simulink library "generator_lib"  (Simulink 7.8)
settings: Solver=ode45  StartTime=0.0  StopTime=10.0  RelTol=1e-3
undefined symbols (not defined in the file): dfilt, DiscIntNeverNeededParam, fdesignblkfcn, gcbh, ph, Ts
libraries: simulink x91, rtio_opalrt_common x84, powerlib x51, simulink_extras x21, discretizing x14, rteventslib x14, dsparch4 x14, powerlib_extras x4
(part 9 of 10)

== system generator_lib/Generator_09112015/GenSet_4MVA_copy1mva/4MVA Generator with  Primary Controllers/Diesel Engine Speed & Voltage Control fast/Excitation/Damping kf.s / (tf.s +1) ==
  note: link disabled
  In : Inport
  1st-Order Discrete Filter : Subsystem  AncestorBlock=|  mask(Discrete 1st-Order Filter){FilterType=Highpass, Tc=damp(2), Ts=Ts, Initialize=on, Vac_Init=[0 0 60], Vdc_Init=damp(1)*v0(2)/damp(2), PlotResponse=off, param1=[1 500 0.1]}
      | powerlib_extras/Discrete 
      | Control Blocks/Discrete
      | 1st-Order
      | Discrete Filter
      mask prompts: FilterType "Filter Type:"; Tc "Time constant (s):"; Ts "Sample time:"; Initialize "Initialize filter states"; Vac_Init "AC initial input: [ Mag  Phase(degrees)  Freq(Hz) ]"; Vdc_Init "DC Initial input:"; PlotResponse "Plot filter response"; param1 "Frequency range(Hz) : [Start  End  Inc.]"
      mask init: same as generator_lib/1MVA Generator/GenSet_900kW_07232015/900kW Generator with  Primary Controllers/Diesel Engine Speed & Voltage Control fast/Excitation/Low Pass Filter 1 / (tr.s +1) (with IC)
      mask StyleString: popup(Lowpass|Highpass),edit,edit,checkbox,edit,edit,checkbox,edit
      mask CallbackString: |||p4=get_param(gcb,'Initialize');if strcmp(p4,'on');visible={'on','on','on','on','on','on','on',get_param(gcb,'PlotResponse')};else;visible={'on','on','on','on','off','off','on',get_param(gcb,'PlotResponse')};end;set_param(gcb,'MaskVisibilities',visible)|||p7=get_param(gcb,'PlotResponse');if strcmp(p7,'on');visible={'on','on','on','on',get_param(gcb,'Initialize'),get_param(gcb,'Initialize'),'on','on'};else;visible={'on','on','on','on',get_param(gcb,'Initialize'),get_param(gcb,'Initialize'),'on','off'};end;set_param(gcb,'MaskVisibilities',visible)|
      mask Display: plot(X,Y);
  Gain : Gain  Gain=damp(1)/damp(2)  SaturateOnIntegerOverflow=on  OutDataTypeStr=Inherit: Same as input  ParamDataTypeStr=Inherit: Same as input
  Out : Outport
  wires:
  1st-Order Discrete Filter/1(Out) -> Out/1
  Gain/1 -> 1st-Order Discrete Filter/1(In)
  In/1 -> Gain/1

== system generator_lib/Generator_09112015/GenSet_4MVA_copy1mva/4MVA Generator with  Primary Controllers/Diesel Engine Speed & Voltage Control fast/Excitation/Exciter  1 / (te.s + ke) ==
  note: link disabled
  In : Inport
  1st order Lowpass : Subsystem  AncestorBlock=|  mask(Discrete 1st-Order Filter){FilterType=Lowpass, Tc=exc(2)/exc(1), Ts=Ts, Initialize=on, Vac_Init=[0.0 0 60], Vdc_Init=v0(2), PlotResponse=off, param1=[1 500 0.1]}
      | powerlib_extras/Discrete 
      | Control Blocks/Discrete
      | 1st-Order
      | Discrete Filter
      mask prompts: FilterType "Filter Type:"; Tc "Time constant (s):"; Ts "Sample time:"; Initialize "Initialize filter states"; Vac_Init "AC initial input: [ Mag  Phase(degrees)  Freq(Hz) ]"; Vdc_Init "DC Initial input:"; PlotResponse "Plot filter response"; param1 "Frequency range(Hz) : [Start  End  Inc.]"
      mask init: same as generator_lib/1MVA Generator/GenSet_900kW_07232015/900kW Generator with  Primary Controllers/Diesel Engine Speed & Voltage Control fast/Excitation/Low Pass Filter 1 / (tr.s +1) (with IC)
      mask StyleString: popup(Lowpass|Highpass),edit,edit,checkbox,edit,edit,checkbox,edit
      mask CallbackString: |||p4=get_param(gcb,'Initialize');if strcmp(p4,'on');visible={'on','on','on','on','on','on','on',get_param(gcb,'PlotResponse')};else;visible={'on','on','on','on','off','off','on',get_param(gcb,'PlotResponse')};end;set_param(gcb,'MaskVisibilities',visible)|||p7=get_param(gcb,'PlotResponse');if strcmp(p7,'on');visible={'on','on','on','on',get_param(gcb,'Initialize'),get_param(gcb,'Initialize'),'on','on'};else;visible={'on','on','on','on',get_param(gcb,'Initialize'),get_param(gcb,'Initialize'),'on','off'};end;set_param(gcb,'MaskVisibilities',visible)|
      mask Display: plot(X,Y);
  Gain : Gain  Gain=1/exc(1)  SaturateOnIntegerOverflow=on  OutDataTypeStr=Inherit: Same as input  ParamDataTypeStr=Inherit: Same as input
  Out : Outport
  wires:
  Gain/1 -> 1st order Lowpass/1(In)
  In/1 -> Gain/1
  1st order Lowpass/1(Out) -> Out/1

== system generator_lib/Generator_09112015/GenSet_4MVA_copy1mva/4MVA Generator with  Primary Controllers/Diesel Engine Speed & Voltage Control fast/Excitation/Lead Lag Compensator tc.s+1 / tb.s+1 ==
  In1 : Inport
  Discrete State-Space : DiscreteStateSpace  A=Ad  B=Bd  C=Cd  D=Dd  X0=x0d  SampleTime=Ts
  Out1 : Outport
  wires:
  In1/1 -> Discrete State-Space/1
  Discrete State-Space/1 -> Out1/1

== system generator_lib/Generator_09112015/GenSet_4MVA_copy1mva/4MVA Generator with  Primary Controllers/Diesel Engine Speed & Voltage Control fast/Excitation/Low Pass Filter 1 / (tr.s +1) (with IC) ==
  In : Inport
  Discrete State-Space : DiscreteStateSpace  A=Ad  B=Bd  C=Cd  D=Dd  X0=x0d  SampleTime=Ts
  Out : Outport  InitialOutput=0
  wires:
  In/1 -> Discrete State-Space/1
  Discrete State-Space/1 -> Out/1

== system generator_lib/Generator_09112015/GenSet_4MVA_copy1mva/4MVA Generator with  Primary Controllers/Diesel Engine Speed & Voltage Control fast/Excitation/Main Regulator ka / (ta.s +1) ==
  note: link disabled
  In : Inport
  1st order Lowpass : Subsystem  AncestorBlock=|  mask(Discrete 1st-Order Filter){FilterType=Lowpass, Tc=reg(2), Ts=Ts, Initialize=on, Vac_Init=[0.0 0 60], Vdc_Init=exc(1)*v0(2), PlotResponse=off, param1=[1 500 0.1]}
      | powerlib_extras/Discrete 
      | Control Blocks/Discrete
      | 1st-Order
      | Discrete Filter
      mask prompts: FilterType "Filter Type:"; Tc "Time constant (s):"; Ts "Sample time:"; Initialize "Initialize filter states"; Vac_Init "AC initial input: [ Mag  Phase(degrees)  Freq(Hz) ]"; Vdc_Init "DC Initial input:"; PlotResponse "Plot filter response"; param1 "Frequency range(Hz) : [Start  End  Inc.]"
      mask init: same as generator_lib/1MVA Generator/GenSet_900kW_07232015/900kW Generator with  Primary Controllers/Diesel Engine Speed & Voltage Control fast/Excitation/Low Pass Filter 1 / (tr.s +1) (with IC)
      mask StyleString: popup(Lowpass|Highpass),edit,edit,checkbox,edit,edit,checkbox,edit
      mask CallbackString: |||p4=get_param(gcb,'Initialize');if strcmp(p4,'on');visible={'on','on','on','on','on','on','on',get_param(gcb,'PlotResponse')};else;visible={'on','on','on','on','off','off','on',get_param(gcb,'PlotResponse')};end;set_param(gcb,'MaskVisibilities',visible)|||p7=get_param(gcb,'PlotResponse');if strcmp(p7,'on');visible={'on','on','on','on',get_param(gcb,'Initialize'),get_param(gcb,'Initialize'),'on','on'};else;visible={'on','on','on','on',get_param(gcb,'Initialize'),get_param(gcb,'Initialize'),'on','off'};end;set_param(gcb,'MaskVisibilities',visible)|
      mask Display: plot(X,Y);
  Gain : Gain  Gain=reg(1)  SaturateOnIntegerOverflow=on  OutDataTypeStr=Inherit: Same as input  ParamDataTypeStr=Inherit: Same as input
  Out : Outport
  wires:
  1st order Lowpass/1(Out) -> Out/1
  In/1 -> Gain/1
  Gain/1 -> 1st order Lowpass/1(In)

== system generator_lib/Generator_09112015/GenSet_4MVA_copy1mva/4MVA Generator with  Primary Controllers/Diesel Engine Speed & Voltage Control fast/Excitation/proportional saturation ==
  Efd : Inport
  Vtf : Inport  Port=2
  Constant : Constant  Value=lim(3)
  Constant1 : Constant  Value=lim(1)
  Constant3 : Constant  Value=0
  Data Type  Conversion{,1..3} (4 alike) : DataTypeConversion  OutDataTypeStr=double  SaturateOnIntegerOverflow=on  RndMeth=Zero
  Logical Operator : Logic
  Logical Operator1 : Logic  Operator=NOT  Inputs=1
  Logical Operator2 : Logic  Operator=NOT  Inputs=1
  Product : Product  SaturateOnIntegerOverflow=on  InputSameDT=on  OutDataTypeStr=Inherit: Same as first input
  Product1 : Product  SaturateOnIntegerOverflow=on  InputSameDT=on  OutDataTypeStr=Inherit: Same as first input
  Product2 : Product  SaturateOnIntegerOverflow=on  InputSameDT=on  OutDataTypeStr=Inherit: Same as first input
  Relational Operator : RelationalOperator  Operator===  InputSameDT=on
  Relational Operator1 : RelationalOperator  Operator=<  InputSameDT=on
  Relational Operator2 : RelationalOperator  Operator=>  InputSameDT=on
  Sum : Sum  SaturateOnIntegerOverflow=on  InputSameDT=on  OutDataTypeStr=Inherit: Same as first input
  Sum1 : Sum  Inputs=+++  SaturateOnIntegerOverflow=on  InputSameDT=on  OutDataTypeStr=Inherit: Same as first input
  Vfdmax : Gain  Gain=lim(2)  SaturateOnIntegerOverflow=on  OutDataTypeStr=Inherit: Same as input  ParamDataTypeStr=Inherit: Same as input
  Vfdmax1 : Gain  Gain=lim(3)  SaturateOnIntegerOverflow=on  OutDataTypeStr=Inherit: Same as input  ParamDataTypeStr=Inherit: Same as input
  Ef : Outport  InitialOutput=0
  wires:
  Data Type  Conversion3/1 -> Vfdmax/1
  Relational Operator/1 -> Data Type  Conversion3/1
  Data Type  Conversion2/1 -> Product2/1
  Logical Operator2/1 -> Data Type  Conversion2/1
  Data Type  Conversion1/1 -> Product1/2
  Logical Operator1/1 -> Data Type  Conversion1/1
  Data Type  Conversion/1 -> Product/2
  Logical Operator/1 -> Data Type  Conversion/1
  Product1/1 -> Sum1/2
  Product2/1 -> Sum1/3
  Product/1 -> Sum1/1
  Sum1/1 -> Ef/1
  Efd/1 -> Product/1, Relational Operator1/1, Relational Operator2/1
  Constant1/1 -> Product1/1, Relational Operator2/2
  Relational Operator1/1 -> Logical Operator/2, Logical Operator2/1
  Relational Operator2/1 -> Logical Operator/1, Logical Operator1/1
  Sum/1 -> Relational Operator1/2, Product2/2
  Vfdmax1/1 -> Sum/1
  Vfdmax/1 -> Sum/2
  Constant3/1 -> Relational Operator/2
  Constant/1 -> Relational Operator/1
  Vtf/1 -> Vfdmax1/1

== system generator_lib/Generator_09142015/GenSet_1MVA_09082015/900kW Generator with  Primary Controllers/Diesel Engine Speed & Voltage Control fast/Excitation/Damping kf.s / (tf.s +1) ==
  note: link disabled
  In : Inport
  1st-Order Discrete Filter : Subsystem  AncestorBlock=|  mask(Discrete 1st-Order Filter){FilterType=Highpass, Tc=damp(2), Ts=Ts, Initialize=on, Vac_Init=[0 0 60], Vdc_Init=damp(1)*v0(2)/damp(2), PlotResponse=off, param1=[1 500 0.1]}
      | powerlib_extras/Discrete 
      | Control Blocks/Discrete
      | 1st-Order
      | Discrete Filter
      mask prompts: FilterType "Filter Type:"; Tc "Time constant (s):"; Ts "Sample time:"; Initialize "Initialize filter states"; Vac_Init "AC initial input: [ Mag  Phase(degrees)  Freq(Hz) ]"; Vdc_Init "DC Initial input:"; PlotResponse "Plot filter response"; param1 "Frequency range(Hz) : [Start  End  Inc.]"
      mask init: same as generator_lib/1MVA Generator/GenSet_900kW_07232015/900kW Generator with  Primary Controllers/Diesel Engine Speed & Voltage Control fast/Excitation/Low Pass Filter 1 / (tr.s +1) (with IC)
      mask StyleString: popup(Lowpass|Highpass),edit,edit,checkbox,edit,edit,checkbox,edit
      mask CallbackString: |||p4=get_param(gcb,'Initialize');if strcmp(p4,'on');visible={'on','on','on','on','on','on','on',get_param(gcb,'PlotResponse')};else;visible={'on','on','on','on','off','off','on',get_param(gcb,'PlotResponse')};end;set_param(gcb,'MaskVisibilities',visible)|||p7=get_param(gcb,'PlotResponse');if strcmp(p7,'on');visible={'on','on','on','on',get_param(gcb,'Initialize'),get_param(gcb,'Initialize'),'on','on'};else;visible={'on','on','on','on',get_param(gcb,'Initialize'),get_param(gcb,'Initialize'),'on','off'};end;set_param(gcb,'MaskVisibilities',visible)|
      mask Display: plot(X,Y);
  Gain : Gain  Gain=damp(1)/damp(2)  SaturateOnIntegerOverflow=on  OutDataTypeStr=Inherit: Same as input  ParamDataTypeStr=Inherit: Same as input
  Out : Outport
  wires:
  In/1 -> Gain/1
  Gain/1 -> 1st-Order Discrete Filter/1(In)
  1st-Order Discrete Filter/1(Out) -> Out/1

== system generator_lib/Generator_09142015/GenSet_1MVA_09082015/900kW Generator with  Primary Controllers/Diesel Engine Speed & Voltage Control fast/Excitation/Exciter  1 / (te.s + ke) ==
  note: link disabled
  In : Inport
  1st order Lowpass : Subsystem  AncestorBlock=|  mask(Discrete 1st-Order Filter){FilterType=Lowpass, Tc=exc(2)/exc(1), Ts=Ts, Initialize=on, Vac_Init=[0.0 0 60], Vdc_Init=v0(2), PlotResponse=off, param1=[1 500 0.1]}
      | powerlib_extras/Discrete 
      | Control Blocks/Discrete
      | 1st-Order
      | Discrete Filter
      mask prompts: FilterType "Filter Type:"; Tc "Time constant (s):"; Ts "Sample time:"; Initialize "Initialize filter states"; Vac_Init "AC initial input: [ Mag  Phase(degrees)  Freq(Hz) ]"; Vdc_Init "DC Initial input:"; PlotResponse "Plot filter response"; param1 "Frequency range(Hz) : [Start  End  Inc.]"
      mask init: same as generator_lib/1MVA Generator/GenSet_900kW_07232015/900kW Generator with  Primary Controllers/Diesel Engine Speed & Voltage Control fast/Excitation/Low Pass Filter 1 / (tr.s +1) (with IC)
      mask StyleString: popup(Lowpass|Highpass),edit,edit,checkbox,edit,edit,checkbox,edit
      mask CallbackString: |||p4=get_param(gcb,'Initialize');if strcmp(p4,'on');visible={'on','on','on','on','on','on','on',get_param(gcb,'PlotResponse')};else;visible={'on','on','on','on','off','off','on',get_param(gcb,'PlotResponse')};end;set_param(gcb,'MaskVisibilities',visible)|||p7=get_param(gcb,'PlotResponse');if strcmp(p7,'on');visible={'on','on','on','on',get_param(gcb,'Initialize'),get_param(gcb,'Initialize'),'on','on'};else;visible={'on','on','on','on',get_param(gcb,'Initialize'),get_param(gcb,'Initialize'),'on','off'};end;set_param(gcb,'MaskVisibilities',visible)|
      mask Display: plot(X,Y);
  Gain : Gain  Gain=1/exc(1)  SaturateOnIntegerOverflow=on  OutDataTypeStr=Inherit: Same as input  ParamDataTypeStr=Inherit: Same as input
  Out : Outport
  wires:
  1st order Lowpass/1(Out) -> Out/1
  In/1 -> Gain/1
  Gain/1 -> 1st order Lowpass/1(In)

== system generator_lib/Generator_09142015/GenSet_1MVA_09082015/900kW Generator with  Primary Controllers/Diesel Engine Speed & Voltage Control fast/Excitation/Lead Lag Compensator tc.s+1 / tb.s+1 ==
  In1 : Inport
  Discrete State-Space : DiscreteStateSpace  A=Ad  B=Bd  C=Cd  D=Dd  X0=x0d  SampleTime=Ts
  Out1 : Outport
  wires:
  Discrete State-Space/1 -> Out1/1
  In1/1 -> Discrete State-Space/1

== system generator_lib/Generator_09142015/GenSet_1MVA_09082015/900kW Generator with  Primary Controllers/Diesel Engine Speed & Voltage Control fast/Excitation/Low Pass Filter 1 / (tr.s +1) (with IC) ==
  In : Inport
  Discrete State-Space : DiscreteStateSpace  A=Ad  B=Bd  C=Cd  D=Dd  X0=x0d  SampleTime=Ts
  Out : Outport  InitialOutput=0
  wires:
  Discrete State-Space/1 -> Out/1
  In/1 -> Discrete State-Space/1

== system generator_lib/Generator_09142015/GenSet_1MVA_09082015/900kW Generator with  Primary Controllers/Diesel Engine Speed & Voltage Control fast/Excitation/Main Regulator ka / (ta.s +1) ==
  note: link disabled
  In : Inport
  1st order Lowpass : Subsystem  AncestorBlock=|  mask(Discrete 1st-Order Filter){FilterType=Lowpass, Tc=reg(2), Ts=Ts, Initialize=on, Vac_Init=[0.0 0 60], Vdc_Init=exc(1)*v0(2), PlotResponse=off, param1=[1 500 0.1]}
      | powerlib_extras/Discrete 
      | Control Blocks/Discrete
      | 1st-Order
      | Discrete Filter
      mask prompts: FilterType "Filter Type:"; Tc "Time constant (s):"; Ts "Sample time:"; Initialize "Initialize filter states"; Vac_Init "AC initial input: [ Mag  Phase(degrees)  Freq(Hz) ]"; Vdc_Init "DC Initial input:"; PlotResponse "Plot filter response"; param1 "Frequency range(Hz) : [Start  End  Inc.]"
      mask init: same as generator_lib/1MVA Generator/GenSet_900kW_07232015/900kW Generator with  Primary Controllers/Diesel Engine Speed & Voltage Control fast/Excitation/Low Pass Filter 1 / (tr.s +1) (with IC)
      mask StyleString: popup(Lowpass|Highpass),edit,edit,checkbox,edit,edit,checkbox,edit
      mask CallbackString: |||p4=get_param(gcb,'Initialize');if strcmp(p4,'on');visible={'on','on','on','on','on','on','on',get_param(gcb,'PlotResponse')};else;visible={'on','on','on','on','off','off','on',get_param(gcb,'PlotResponse')};end;set_param(gcb,'MaskVisibilities',visible)|||p7=get_param(gcb,'PlotResponse');if strcmp(p7,'on');visible={'on','on','on','on',get_param(gcb,'Initialize'),get_param(gcb,'Initialize'),'on','on'};else;visible={'on','on','on','on',get_param(gcb,'Initialize'),get_param(gcb,'Initialize'),'on','off'};end;set_param(gcb,'MaskVisibilities',visible)|
      mask Display: plot(X,Y);
  Gain : Gain  Gain=reg(1)  SaturateOnIntegerOverflow=on  OutDataTypeStr=Inherit: Same as input  ParamDataTypeStr=Inherit: Same as input
  Out : Outport
  wires:
  Gain/1 -> 1st order Lowpass/1(In)
  In/1 -> Gain/1
  1st order Lowpass/1(Out) -> Out/1

== system generator_lib/Generator_09142015/GenSet_1MVA_09082015/900kW Generator with  Primary Controllers/Diesel Engine Speed & Voltage Control fast/Excitation/proportional saturation ==
  Efd : Inport
  Vtf : Inport  Port=2
  Constant : Constant  Value=lim(3)
  Constant1 : Constant  Value=lim(1)
  Constant3 : Constant  Value=0
  Data Type  Conversion{,1..3} (4 alike) : DataTypeConversion  OutDataTypeStr=double  SaturateOnIntegerOverflow=on  RndMeth=Zero
  Logical Operator : Logic
  Logical Operator1 : Logic  Operator=NOT  Inputs=1
  Logical Operator2 : Logic  Operator=NOT  Inputs=1
  Product : Product  SaturateOnIntegerOverflow=on  InputSameDT=on  OutDataTypeStr=Inherit: Same as first input
  Product1 : Product  SaturateOnIntegerOverflow=on  InputSameDT=on  OutDataTypeStr=Inherit: Same as first input
  Product2 : Product  SaturateOnIntegerOverflow=on  InputSameDT=on  OutDataTypeStr=Inherit: Same as first input
  Relational Operator : RelationalOperator  Operator===  InputSameDT=on
  Relational Operator1 : RelationalOperator  Operator=<  InputSameDT=on
  Relational Operator2 : RelationalOperator  Operator=>  InputSameDT=on
  Sum : Sum  SaturateOnIntegerOverflow=on  InputSameDT=on  OutDataTypeStr=Inherit: Same as first input
  Sum1 : Sum  Inputs=+++  SaturateOnIntegerOverflow=on  InputSameDT=on  OutDataTypeStr=Inherit: Same as first input
  Vfdmax : Gain  Gain=lim(2)  SaturateOnIntegerOverflow=on  OutDataTypeStr=Inherit: Same as input  ParamDataTypeStr=Inherit: Same as input
  Vfdmax1 : Gain  Gain=lim(3)  SaturateOnIntegerOverflow=on  OutDataTypeStr=Inherit: Same as input  ParamDataTypeStr=Inherit: Same as input
  Ef : Outport  InitialOutput=0
  wires:
  Vtf/1 -> Vfdmax1/1
  Constant/1 -> Relational Operator/1
  Constant3/1 -> Relational Operator/2
  Vfdmax/1 -> Sum/2
  Vfdmax1/1 -> Sum/1
  Sum/1 -> Product2/2, Relational Operator1/2
  Relational Operator2/1 -> Logical Operator1/1, Logical Operator/1
  Relational Operator1/1 -> Logical Operator2/1, Logical Operator/2
  Constant1/1 -> Relational Operator2/2, Product1/1
  Efd/1 -> Relational Operator2/1, Relational Operator1/1, Product/1
  Sum1/1 -> Ef/1
  Product/1 -> Sum1/1
  Product2/1 -> Sum1/3
  Product1/1 -> Sum1/2
  Logical Operator/1 -> Data Type  Conversion/1
  Data Type  Conversion/1 -> Product/2
  Logical Operator1/1 -> Data Type  Conversion1/1
  Data Type  Conversion1/1 -> Product1/2
  Logical Operator2/1 -> Data Type  Conversion2/1
  Data Type  Conversion2/1 -> Product2/1
  Relational Operator/1 -> Data Type  Conversion3/1
  Data Type  Conversion3/1 -> Vfdmax/1

== system generator_lib/Generator_09142015/GenSet_4MVA_09142015/4MVA Generator with  Primary Controllers/Diesel Engine Speed & Voltage Control fast/Excitation/Damping kf.s / (tf.s +1) ==
  note: link disabled
  In : Inport
  1st-Order Discrete Filter : Subsystem  AncestorBlock=|  mask(Discrete 1st-Order Filter){FilterType=Highpass, Tc=damp(2), Ts=Ts, Initialize=on, Vac_Init=[0 0 60], Vdc_Init=damp(1)*v0(2)/damp(2), PlotResponse=off, param1=[1 500 0.1]}
      | powerlib_extras/Discrete 
      | Control Blocks/Discrete
      | 1st-Order
      | Discrete Filter
      mask prompts: FilterType "Filter Type:"; Tc "Time constant (s):"; Ts "Sample time:"; Initialize "Initialize filter states"; Vac_Init "AC initial input: [ Mag  Phase(degrees)  Freq(Hz) ]"; Vdc_Init "DC Initial input:"; PlotResponse "Plot filter response"; param1 "Frequency range(Hz) : [Start  End  Inc.]"
      mask init: same as generator_lib/1MVA Generator/GenSet_900kW_07232015/900kW Generator with  Primary Controllers/Diesel Engine Speed & Voltage Control fast/Excitation/Low Pass Filter 1 / (tr.s +1) (with IC)
      mask StyleString: popup(Lowpass|Highpass),edit,edit,checkbox,edit,edit,checkbox,edit
      mask CallbackString: |||p4=get_param(gcb,'Initialize');if strcmp(p4,'on');visible={'on','on','on','on','on','on','on',get_param(gcb,'PlotResponse')};else;visible={'on','on','on','on','off','off','on',get_param(gcb,'PlotResponse')};end;set_param(gcb,'MaskVisibilities',visible)|||p7=get_param(gcb,'PlotResponse');if strcmp(p7,'on');visible={'on','on','on','on',get_param(gcb,'Initialize'),get_param(gcb,'Initialize'),'on','on'};else;visible={'on','on','on','on',get_param(gcb,'Initialize'),get_param(gcb,'Initialize'),'on','off'};end;set_param(gcb,'MaskVisibilities',visible)|
      mask Display: plot(X,Y);
  Gain : Gain  Gain=damp(1)/damp(2)  SaturateOnIntegerOverflow=on  OutDataTypeStr=Inherit: Same as input  ParamDataTypeStr=Inherit: Same as input
  Out : Outport
  wires:
  In/1 -> Gain/1
  Gain/1 -> 1st-Order Discrete Filter/1(In)
  1st-Order Discrete Filter/1(Out) -> Out/1

== system generator_lib/Generator_09142015/GenSet_4MVA_09142015/4MVA Generator with  Primary Controllers/Diesel Engine Speed & Voltage Control fast/Excitation/Exciter  1 / (te.s + ke) ==
  note: link disabled
  In : Inport
  1st order Lowpass : Subsystem  AncestorBlock=|  mask(Discrete 1st-Order Filter){FilterType=Lowpass, Tc=exc(2)/exc(1), Ts=Ts, Initialize=on, Vac_Init=[0.0 0 60], Vdc_Init=v0(2), PlotResponse=off, param1=[1 500 0.1]}
      | powerlib_extras/Discrete 
      | Control Blocks/Discrete
      | 1st-Order
      | Discrete Filter
      mask prompts: FilterType "Filter Type:"; Tc "Time constant (s):"; Ts "Sample time:"; Initialize "Initialize filter states"; Vac_Init "AC initial input: [ Mag  Phase(degrees)  Freq(Hz) ]"; Vdc_Init "DC Initial input:"; PlotResponse "Plot filter response"; param1 "Frequency range(Hz) : [Start  End  Inc.]"
      mask init: same as generator_lib/1MVA Generator/GenSet_900kW_07232015/900kW Generator with  Primary Controllers/Diesel Engine Speed & Voltage Control fast/Excitation/Low Pass Filter 1 / (tr.s +1) (with IC)
      mask StyleString: popup(Lowpass|Highpass),edit,edit,checkbox,edit,edit,checkbox,edit
      mask CallbackString: |||p4=get_param(gcb,'Initialize');if strcmp(p4,'on');visible={'on','on','on','on','on','on','on',get_param(gcb,'PlotResponse')};else;visible={'on','on','on','on','off','off','on',get_param(gcb,'PlotResponse')};end;set_param(gcb,'MaskVisibilities',visible)|||p7=get_param(gcb,'PlotResponse');if strcmp(p7,'on');visible={'on','on','on','on',get_param(gcb,'Initialize'),get_param(gcb,'Initialize'),'on','on'};else;visible={'on','on','on','on',get_param(gcb,'Initialize'),get_param(gcb,'Initialize'),'on','off'};end;set_param(gcb,'MaskVisibilities',visible)|
      mask Display: plot(X,Y);
  Gain : Gain  Gain=1/exc(1)  SaturateOnIntegerOverflow=on  OutDataTypeStr=Inherit: Same as input  ParamDataTypeStr=Inherit: Same as input
  Out : Outport
  wires:
  1st order Lowpass/1(Out) -> Out/1
  In/1 -> Gain/1
  Gain/1 -> 1st order Lowpass/1(In)

== system generator_lib/Generator_09142015/GenSet_4MVA_09142015/4MVA Generator with  Primary Controllers/Diesel Engine Speed & Voltage Control fast/Excitation/Lead Lag Compensator tc.s+1 / tb.s+1 ==
  In1 : Inport
  Discrete State-Space : DiscreteStateSpace  A=Ad  B=Bd  C=Cd  D=Dd  X0=x0d  SampleTime=Ts
  Out1 : Outport
  wires:
  Discrete State-Space/1 -> Out1/1
  In1/1 -> Discrete State-Space/1

== system generator_lib/Generator_09142015/GenSet_4MVA_09142015/4MVA Generator with  Primary Controllers/Diesel Engine Speed & Voltage Control fast/Excitation/Low Pass Filter 1 / (tr.s +1) (with IC) ==
  In : Inport
  Discrete State-Space : DiscreteStateSpace  A=Ad  B=Bd  C=Cd  D=Dd  X0=x0d  SampleTime=Ts
  Out : Outport  InitialOutput=0
  wires:
  Discrete State-Space/1 -> Out/1
  In/1 -> Discrete State-Space/1

== system generator_lib/Generator_09142015/GenSet_4MVA_09142015/4MVA Generator with  Primary Controllers/Diesel Engine Speed & Voltage Control fast/Excitation/Main Regulator ka / (ta.s +1) ==
  note: link disabled
  In : Inport
  1st order Lowpass : Subsystem  AncestorBlock=|  mask(Discrete 1st-Order Filter){FilterType=Lowpass, Tc=reg(2), Ts=Ts, Initialize=on, Vac_Init=[0.0 0 60], Vdc_Init=exc(1)*v0(2), PlotResponse=off, param1=[1 500 0.1]}
      | powerlib_extras/Discrete 
      | Control Blocks/Discrete
      | 1st-Order
      | Discrete Filter
      mask prompts: FilterType "Filter Type:"; Tc "Time constant (s):"; Ts "Sample time:"; Initialize "Initialize filter states"; Vac_Init "AC initial input: [ Mag  Phase(degrees)  Freq(Hz) ]"; Vdc_Init "DC Initial input:"; PlotResponse "Plot filter response"; param1 "Frequency range(Hz) : [Start  End  Inc.]"
      mask init: same as generator_lib/1MVA Generator/GenSet_900kW_07232015/900kW Generator with  Primary Controllers/Diesel Engine Speed & Voltage Control fast/Excitation/Low Pass Filter 1 / (tr.s +1) (with IC)
      mask StyleString: popup(Lowpass|Highpass),edit,edit,checkbox,edit,edit,checkbox,edit
      mask CallbackString: |||p4=get_param(gcb,'Initialize');if strcmp(p4,'on');visible={'on','on','on','on','on','on','on',get_param(gcb,'PlotResponse')};else;visible={'on','on','on','on','off','off','on',get_param(gcb,'PlotResponse')};end;set_param(gcb,'MaskVisibilities',visible)|||p7=get_param(gcb,'PlotResponse');if strcmp(p7,'on');visible={'on','on','on','on',get_param(gcb,'Initialize'),get_param(gcb,'Initialize'),'on','on'};else;visible={'on','on','on','on',get_param(gcb,'Initialize'),get_param(gcb,'Initialize'),'on','off'};end;set_param(gcb,'MaskVisibilities',visible)|
      mask Display: plot(X,Y);
  Gain : Gain  Gain=reg(1)  SaturateOnIntegerOverflow=on  OutDataTypeStr=Inherit: Same as input  ParamDataTypeStr=Inherit: Same as input
  Out : Outport
  wires:
  Gain/1 -> 1st order Lowpass/1(In)
  In/1 -> Gain/1
  1st order Lowpass/1(Out) -> Out/1

== system generator_lib/Generator_09142015/GenSet_4MVA_09142015/4MVA Generator with  Primary Controllers/Diesel Engine Speed & Voltage Control fast/Excitation/proportional saturation ==
  Efd : Inport
  Vtf : Inport  Port=2
  Constant : Constant  Value=lim(3)
  Constant1 : Constant  Value=lim(1)
  Constant3 : Constant  Value=0
  Data Type  Conversion{,1..3} (4 alike) : DataTypeConversion  OutDataTypeStr=double  SaturateOnIntegerOverflow=on  RndMeth=Zero
  Logical Operator : Logic
  Logical Operator1 : Logic  Operator=NOT  Inputs=1
  Logical Operator2 : Logic  Operator=NOT  Inputs=1
  Product : Product  SaturateOnIntegerOverflow=on  InputSameDT=on  OutDataTypeStr=Inherit: Same as first input
  Product1 : Product  SaturateOnIntegerOverflow=on  InputSameDT=on  OutDataTypeStr=Inherit: Same as first input
  Product2 : Product  SaturateOnIntegerOverflow=on  InputSameDT=on  OutDataTypeStr=Inherit: Same as first input
  Relational Operator : RelationalOperator  Operator===  InputSameDT=on
  Relational Operator1 : RelationalOperator  Operator=<  InputSameDT=on
  Relational Operator2 : RelationalOperator  Operator=>  InputSameDT=on
  Sum : Sum  SaturateOnIntegerOverflow=on  InputSameDT=on  OutDataTypeStr=Inherit: Same as first input
  Sum1 : Sum  Inputs=+++  SaturateOnIntegerOverflow=on  InputSameDT=on  OutDataTypeStr=Inherit: Same as first input
  Vfdmax : Gain  Gain=lim(2)  SaturateOnIntegerOverflow=on  OutDataTypeStr=Inherit: Same as input  ParamDataTypeStr=Inherit: Same as input
  Vfdmax1 : Gain  Gain=lim(3)  SaturateOnIntegerOverflow=on  OutDataTypeStr=Inherit: Same as input  ParamDataTypeStr=Inherit: Same as input
  Ef : Outport  InitialOutput=0
  wires:
  Vtf/1 -> Vfdmax1/1
  Constant/1 -> Relational Operator/1
  Constant3/1 -> Relational Operator/2
  Vfdmax/1 -> Sum/2
  Vfdmax1/1 -> Sum/1
  Sum/1 -> Product2/2, Relational Operator1/2
  Relational Operator2/1 -> Logical Operator1/1, Logical Operator/1
  Relational Operator1/1 -> Logical Operator2/1, Logical Operator/2
  Constant1/1 -> Relational Operator2/2, Product1/1
  Efd/1 -> Relational Operator2/1, Relational Operator1/1, Product/1
  Sum1/1 -> Ef/1
  Product/1 -> Sum1/1
  Product2/1 -> Sum1/3
  Product1/1 -> Sum1/2
  Logical Operator/1 -> Data Type  Conversion/1
  Data Type  Conversion/1 -> Product/2
  Logical Operator1/1 -> Data Type  Conversion1/1
  Data Type  Conversion1/1 -> Product1/2
  Logical Operator2/1 -> Data Type  Conversion2/1
  Data Type  Conversion2/1 -> Product2/1
  Relational Operator/1 -> Data Type  Conversion3/1
  Data Type  Conversion3/1 -> Vfdmax/1

== system generator_lib/Generator_09152015/GenSet_1MVA_09082015/900kW Generator with  Primary Controllers/Diesel Engine Speed & Voltage Control fast/Excitation/Damping kf.s / (tf.s +1) ==
  note: link disabled
  In : Inport
  1st-Order Discrete Filter : Subsystem  AncestorBlock=|  mask(Discrete 1st-Order Filter){FilterType=Highpass, Tc=damp(2), Ts=Ts, Initialize=on, Vac_Init=[0 0 60], Vdc_Init=damp(1)*v0(2)/damp(2), PlotResponse=off, param1=[1 500 0.1]}
      | powerlib_extras/Discrete 
      | Control Blocks/Discrete
      | 1st-Order
      | Discrete Filter
      mask prompts: FilterType "Filter Type:"; Tc "Time constant (s):"; Ts "Sample time:"; Initialize "Initialize filter states"; Vac_Init "AC initial input: [ Mag  Phase(degrees)  Freq(Hz) ]"; Vdc_Init "DC Initial input:"; PlotResponse "Plot filter response"; param1 "Frequency range(Hz) : [Start  End  Inc.]"
      mask init: same as generator_lib/1MVA Generator/GenSet_900kW_07232015/900kW Generator with  Primary Controllers/Diesel Engine Speed & Voltage Control fast/Excitation/Low Pass Filter 1 / (tr.s +1) (with IC)
      mask StyleString: popup(Lowpass|Highpass),edit,edit,checkbox,edit,edit,checkbox,edit
      mask CallbackString: |||p4=get_param(gcb,'Initialize');if strcmp(p4,'on');visible={'on','on','on','on','on','on','on',get_param(gcb,'PlotResponse')};else;visible={'on','on','on','on','off','off','on',get_param(gcb,'PlotResponse')};end;set_param(gcb,'MaskVisibilities',visible)|||p7=get_param(gcb,'PlotResponse');if strcmp(p7,'on');visible={'on','on','on','on',get_param(gcb,'Initialize'),get_param(gcb,'Initialize'),'on','on'};else;visible={'on','on','on','on',get_param(gcb,'Initialize'),get_param(gcb,'Initialize'),'on','off'};end;set_param(gcb,'MaskVisibilities',visible)|
      mask Display: plot(X,Y);
  Gain : Gain  Gain=damp(1)/damp(2)  SaturateOnIntegerOverflow=on  OutDataTypeStr=Inherit: Same as input  ParamDataTypeStr=Inherit: Same as input
  Out : Outport
  wires:
  In/1 -> Gain/1
  Gain/1 -> 1st-Order Discrete Filter/1(In)
  1st-Order Discrete Filter/1(Out) -> Out/1

== system generator_lib/Generator_09152015/GenSet_1MVA_09082015/900kW Generator with  Primary Controllers/Diesel Engine Speed & Voltage Control fast/Excitation/Exciter  1 / (te.s + ke) ==
  note: link disabled
  In : Inport
  1st order Lowpass : Subsystem  AncestorBlock=|  mask(Discrete 1st-Order Filter){FilterType=Lowpass, Tc=exc(2)/exc(1), Ts=Ts, Initialize=on, Vac_Init=[0.0 0 60], Vdc_Init=v0(2), PlotResponse=off, param1=[1 500 0.1]}
      | powerlib_extras/Discrete 
      | Control Blocks/Discrete
      | 1st-Order
      | Discrete Filter
      mask prompts: FilterType "Filter Type:"; Tc "Time constant (s):"; Ts "Sample time:"; Initialize "Initialize filter states"; Vac_Init "AC initial input: [ Mag  Phase(degrees)  Freq(Hz) ]"; Vdc_Init "DC Initial input:"; PlotResponse "Plot filter response"; param1 "Frequency range(Hz) : [Start  End  Inc.]"
      mask init: same as generator_lib/1MVA Generator/GenSet_900kW_07232015/900kW Generator with  Primary Controllers/Diesel Engine Speed & Voltage Control fast/Excitation/Low Pass Filter 1 / (tr.s +1) (with IC)
      mask StyleString: popup(Lowpass|Highpass),edit,edit,checkbox,edit,edit,checkbox,edit
      mask CallbackString: |||p4=get_param(gcb,'Initialize');if strcmp(p4,'on');visible={'on','on','on','on','on','on','on',get_param(gcb,'PlotResponse')};else;visible={'on','on','on','on','off','off','on',get_param(gcb,'PlotResponse')};end;set_param(gcb,'MaskVisibilities',visible)|||p7=get_param(gcb,'PlotResponse');if strcmp(p7,'on');visible={'on','on','on','on',get_param(gcb,'Initialize'),get_param(gcb,'Initialize'),'on','on'};else;visible={'on','on','on','on',get_param(gcb,'Initialize'),get_param(gcb,'Initialize'),'on','off'};end;set_param(gcb,'MaskVisibilities',visible)|
      mask Display: plot(X,Y);
  Gain : Gain  Gain=1/exc(1)  SaturateOnIntegerOverflow=on  OutDataTypeStr=Inherit: Same as input  ParamDataTypeStr=Inherit: Same as input
  Out : Outport
  wires:
  1st order Lowpass/1(Out) -> Out/1
  In/1 -> Gain/1
  Gain/1 -> 1st order Lowpass/1(In)

== system generator_lib/Generator_09152015/GenSet_1MVA_09082015/900kW Generator with  Primary Controllers/Diesel Engine Speed & Voltage Control fast/Excitation/Lead Lag Compensator tc.s+1 / tb.s+1 ==
  In1 : Inport
  Discrete State-Space : DiscreteStateSpace  A=Ad  B=Bd  C=Cd  D=Dd  X0=x0d  SampleTime=Ts
  Out1 : Outport
  wires:
  Discrete State-Space/1 -> Out1/1
  In1/1 -> Discrete State-Space/1

== system generator_lib/Generator_09152015/GenSet_1MVA_09082015/900kW Generator with  Primary Controllers/Diesel Engine Speed & Voltage Control fast/Excitation/Low Pass Filter 1 / (tr.s +1) (with IC) ==
  In : Inport
  Discrete State-Space : DiscreteStateSpace  A=Ad  B=Bd  C=Cd  D=Dd  X0=x0d  SampleTime=Ts
  Out : Outport  InitialOutput=0
  wires:
  Discrete State-Space/1 -> Out/1
  In/1 -> Discrete State-Space/1

== system generator_lib/Generator_09152015/GenSet_1MVA_09082015/900kW Generator with  Primary Controllers/Diesel Engine Speed & Voltage Control fast/Excitation/Main Regulator ka / (ta.s +1) ==
  note: link disabled
  In : Inport
  1st order Lowpass : Subsystem  AncestorBlock=|  mask(Discrete 1st-Order Filter){FilterType=Lowpass, Tc=reg(2), Ts=Ts, Initialize=on, Vac_Init=[0.0 0 60], Vdc_Init=exc(1)*v0(2), PlotResponse=off, param1=[1 500 0.1]}
      | powerlib_extras/Discrete 
      | Control Blocks/Discrete
      | 1st-Order
      | Discrete Filter
      mask prompts: FilterType "Filter Type:"; Tc "Time constant (s):"; Ts "Sample time:"; Initialize "Initialize filter states"; Vac_Init "AC initial input: [ Mag  Phase(degrees)  Freq(Hz) ]"; Vdc_Init "DC Initial input:"; PlotResponse "Plot filter response"; param1 "Frequency range(Hz) : [Start  End  Inc.]"
      mask init: same as generator_lib/1MVA Generator/GenSet_900kW_07232015/900kW Generator with  Primary Controllers/Diesel Engine Speed & Voltage Control fast/Excitation/Low Pass Filter 1 / (tr.s +1) (with IC)
      mask StyleString: popup(Lowpass|Highpass),edit,edit,checkbox,edit,edit,checkbox,edit
      mask CallbackString: |||p4=get_param(gcb,'Initialize');if strcmp(p4,'on');visible={'on','on','on','on','on','on','on',get_param(gcb,'PlotResponse')};else;visible={'on','on','on','on','off','off','on',get_param(gcb,'PlotResponse')};end;set_param(gcb,'MaskVisibilities',visible)|||p7=get_param(gcb,'PlotResponse');if strcmp(p7,'on');visible={'on','on','on','on',get_param(gcb,'Initialize'),get_param(gcb,'Initialize'),'on','on'};else;visible={'on','on','on','on',get_param(gcb,'Initialize'),get_param(gcb,'Initialize'),'on','off'};end;set_param(gcb,'MaskVisibilities',visible)|
      mask Display: plot(X,Y);
  Gain : Gain  Gain=reg(1)  SaturateOnIntegerOverflow=on  OutDataTypeStr=Inherit: Same as input  ParamDataTypeStr=Inherit: Same as input
  Out : Outport
  wires:
  Gain/1 -> 1st order Lowpass/1(In)
  In/1 -> Gain/1
  1st order Lowpass/1(Out) -> Out/1

== system generator_lib/Generator_09152015/GenSet_1MVA_09082015/900kW Generator with  Primary Controllers/Diesel Engine Speed & Voltage Control fast/Excitation/proportional saturation ==
  Efd : Inport
  Vtf : Inport  Port=2
  Constant : Constant  Value=lim(3)
  Constant1 : Constant  Value=lim(1)
  Constant3 : Constant  Value=0
  Data Type  Conversion{,1..3} (4 alike) : DataTypeConversion  OutDataTypeStr=double  SaturateOnIntegerOverflow=on  RndMeth=Zero
  Logical Operator : Logic
  Logical Operator1 : Logic  Operator=NOT  Inputs=1
  Logical Operator2 : Logic  Operator=NOT  Inputs=1
  Product : Product  SaturateOnIntegerOverflow=on  InputSameDT=on  OutDataTypeStr=Inherit: Same as first input
  Product1 : Product  SaturateOnIntegerOverflow=on  InputSameDT=on  OutDataTypeStr=Inherit: Same as first input
  Product2 : Product  SaturateOnIntegerOverflow=on  InputSameDT=on  OutDataTypeStr=Inherit: Same as first input
  Relational Operator : RelationalOperator  Operator===  InputSameDT=on
  Relational Operator1 : RelationalOperator  Operator=<  InputSameDT=on
  Relational Operator2 : RelationalOperator  Operator=>  InputSameDT=on
  Sum : Sum  SaturateOnIntegerOverflow=on  InputSameDT=on  OutDataTypeStr=Inherit: Same as first input
  Sum1 : Sum  Inputs=+++  SaturateOnIntegerOverflow=on  InputSameDT=on  OutDataTypeStr=Inherit: Same as first input
  Vfdmax : Gain  Gain=lim(2)  SaturateOnIntegerOverflow=on  OutDataTypeStr=Inherit: Same as input  ParamDataTypeStr=Inherit: Same as input
  Vfdmax1 : Gain  Gain=lim(3)  SaturateOnIntegerOverflow=on  OutDataTypeStr=Inherit: Same as input  ParamDataTypeStr=Inherit: Same as input
  Ef : Outport  InitialOutput=0
  wires:
  Vtf/1 -> Vfdmax1/1
  Constant/1 -> Relational Operator/1
  Constant3/1 -> Relational Operator/2
  Vfdmax/1 -> Sum/2
  Vfdmax1/1 -> Sum/1
  Sum/1 -> Product2/2, Relational Operator1/2
  Relational Operator2/1 -> Logical Operator1/1, Logical Operator/1
  Relational Operator1/1 -> Logical Operator2/1, Logical Operator/2
  Constant1/1 -> Relational Operator2/2, Product1/1
  Efd/1 -> Relational Operator2/1, Relational Operator1/1, Product/1
  Sum1/1 -> Ef/1
  Product/1 -> Sum1/1
  Product2/1 -> Sum1/3
  Product1/1 -> Sum1/2
  Logical Operator/1 -> Data Type  Conversion/1
  Data Type  Conversion/1 -> Product/2
  Logical Operator1/1 -> Data Type  Conversion1/1
  Data Type  Conversion1/1 -> Product1/2
  Logical Operator2/1 -> Data Type  Conversion2/1
  Data Type  Conversion2/1 -> Product2/1
  Relational Operator/1 -> Data Type  Conversion3/1
  Data Type  Conversion3/1 -> Vfdmax/1

== system generator_lib/Generator_09152015/GenSet_4MVA_09142015/4MVA Generator with  Primary Controllers/Diesel Engine Speed & Voltage Control fast/Excitation/Damping kf.s / (tf.s +1) ==
  note: link disabled
  In : Inport
  1st-Order Discrete Filter : Subsystem  AncestorBlock=|  mask(Discrete 1st-Order Filter){FilterType=Highpass, Tc=damp(2), Ts=Ts, Initialize=on, Vac_Init=[0 0 60], Vdc_Init=damp(1)*v0(2)/damp(2), PlotResponse=off, param1=[1 500 0.1]}
      | powerlib_extras/Discrete 
      | Control Blocks/Discrete
      | 1st-Order
      | Discrete Filter
      mask prompts: FilterType "Filter Type:"; Tc "Time constant (s):"; Ts "Sample time:"; Initialize "Initialize filter states"; Vac_Init "AC initial input: [ Mag  Phase(degrees)  Freq(Hz) ]"; Vdc_Init "DC Initial input:"; PlotResponse "Plot filter response"; param1 "Frequency range(Hz) : [Start  End  Inc.]"
      mask init: same as generator_lib/1MVA Generator/GenSet_900kW_07232015/900kW Generator with  Primary Controllers/Diesel Engine Speed & Voltage Control fast/Excitation/Low Pass Filter 1 / (tr.s +1) (with IC)
      mask StyleString: popup(Lowpass|Highpass),edit,edit,checkbox,edit,edit,checkbox,edit
      mask CallbackString: |||p4=get_param(gcb,'Initialize');if strcmp(p4,'on');visible={'on','on','on','on','on','on','on',get_param(gcb,'PlotResponse')};else;visible={'on','on','on','on','off','off','on',get_param(gcb,'PlotResponse')};end;set_param(gcb,'MaskVisibilities',visible)|||p7=get_param(gcb,'PlotResponse');if strcmp(p7,'on');visible={'on','on','on','on',get_param(gcb,'Initialize'),get_param(gcb,'Initialize'),'on','on'};else;visible={'on','on','on','on',get_param(gcb,'Initialize'),get_param(gcb,'Initialize'),'on','off'};end;set_param(gcb,'MaskVisibilities',visible)|
      mask Display: plot(X,Y);
  Gain : Gain  Gain=damp(1)/damp(2)  SaturateOnIntegerOverflow=on  OutDataTypeStr=Inherit: Same as input  ParamDataTypeStr=Inherit: Same as input
  Out : Outport
  wires:
  In/1 -> Gain/1
  Gain/1 -> 1st-Order Discrete Filter/1(In)
  1st-Order Discrete Filter/1(Out) -> Out/1

== system generator_lib/Generator_09152015/GenSet_4MVA_09142015/4MVA Generator with  Primary Controllers/Diesel Engine Speed & Voltage Control fast/Excitation/Exciter  1 / (te.s + ke) ==
  note: link disabled
  In : Inport
  1st order Lowpass : Subsystem  AncestorBlock=|  mask(Discrete 1st-Order Filter){FilterType=Lowpass, Tc=exc(2)/exc(1), Ts=Ts, Initialize=on, Vac_Init=[0.0 0 60], Vdc_Init=v0(2), PlotResponse=off, param1=[1 500 0.1]}
      | powerlib_extras/Discrete 
      | Control Blocks/Discrete
      | 1st-Order
      | Discrete Filter
      mask prompts: FilterType "Filter Type:"; Tc "Time constant (s):"; Ts "Sample time:"; Initialize "Initialize filter states"; Vac_Init "AC initial input: [ Mag  Phase(degrees)  Freq(Hz) ]"; Vdc_Init "DC Initial input:"; PlotResponse "Plot filter response"; param1 "Frequency range(Hz) : [Start  End  Inc.]"
      mask init: same as generator_lib/1MVA Generator/GenSet_900kW_07232015/900kW Generator with  Primary Controllers/Diesel Engine Speed & Voltage Control fast/Excitation/Low Pass Filter 1 / (tr.s +1) (with IC)
      mask StyleString: popup(Lowpass|Highpass),edit,edit,checkbox,edit,edit,checkbox,edit
      mask CallbackString: |||p4=get_param(gcb,'Initialize');if strcmp(p4,'on');visible={'on','on','on','on','on','on','on',get_param(gcb,'PlotResponse')};else;visible={'on','on','on','on','off','off','on',get_param(gcb,'PlotResponse')};end;set_param(gcb,'MaskVisibilities',visible)|||p7=get_param(gcb,'PlotResponse');if strcmp(p7,'on');visible={'on','on','on','on',get_param(gcb,'Initialize'),get_param(gcb,'Initialize'),'on','on'};else;visible={'on','on','on','on',get_param(gcb,'Initialize'),get_param(gcb,'Initialize'),'on','off'};end;set_param(gcb,'MaskVisibilities',visible)|
      mask Display: plot(X,Y);
  Gain : Gain  Gain=1/exc(1)  SaturateOnIntegerOverflow=on  OutDataTypeStr=Inherit: Same as input  ParamDataTypeStr=Inherit: Same as input
  Out : Outport
  wires:
  1st order Lowpass/1(Out) -> Out/1
  In/1 -> Gain/1
  Gain/1 -> 1st order Lowpass/1(In)

== system generator_lib/Generator_09152015/GenSet_4MVA_09142015/4MVA Generator with  Primary Controllers/Diesel Engine Speed & Voltage Control fast/Excitation/Lead Lag Compensator tc.s+1 / tb.s+1 ==
  In1 : Inport
  Discrete State-Space : DiscreteStateSpace  A=Ad  B=Bd  C=Cd  D=Dd  X0=x0d  SampleTime=Ts
  Out1 : Outport
  wires:
  Discrete State-Space/1 -> Out1/1
  In1/1 -> Discrete State-Space/1

== system generator_lib/Generator_09152015/GenSet_4MVA_09142015/4MVA Generator with  Primary Controllers/Diesel Engine Speed & Voltage Control fast/Excitation/Low Pass Filter 1 / (tr.s +1) (with IC) ==
  In : Inport
  Discrete State-Space : DiscreteStateSpace  A=Ad  B=Bd  C=Cd  D=Dd  X0=x0d  SampleTime=Ts
  Out : Outport  InitialOutput=0
  wires:
  Discrete State-Space/1 -> Out/1
  In/1 -> Discrete State-Space/1

== system generator_lib/Generator_09152015/GenSet_4MVA_09142015/4MVA Generator with  Primary Controllers/Diesel Engine Speed & Voltage Control fast/Excitation/Main Regulator ka / (ta.s +1) ==
  note: link disabled
  In : Inport
  1st order Lowpass : Subsystem  AncestorBlock=|  mask(Discrete 1st-Order Filter){FilterType=Lowpass, Tc=reg(2), Ts=Ts, Initialize=on, Vac_Init=[0.0 0 60], Vdc_Init=exc(1)*v0(2), PlotResponse=off, param1=[1 500 0.1]}
      | powerlib_extras/Discrete 
      | Control Blocks/Discrete
      | 1st-Order
      | Discrete Filter
      mask prompts: FilterType "Filter Type:"; Tc "Time constant (s):"; Ts "Sample time:"; Initialize "Initialize filter states"; Vac_Init "AC initial input: [ Mag  Phase(degrees)  Freq(Hz) ]"; Vdc_Init "DC Initial input:"; PlotResponse "Plot filter response"; param1 "Frequency range(Hz) : [Start  End  Inc.]"
      mask init: same as generator_lib/1MVA Generator/GenSet_900kW_07232015/900kW Generator with  Primary Controllers/Diesel Engine Speed & Voltage Control fast/Excitation/Low Pass Filter 1 / (tr.s +1) (with IC)
      mask StyleString: popup(Lowpass|Highpass),edit,edit,checkbox,edit,edit,checkbox,edit
      mask CallbackString: |||p4=get_param(gcb,'Initialize');if strcmp(p4,'on');visible={'on','on','on','on','on','on','on',get_param(gcb,'PlotResponse')};else;visible={'on','on','on','on','off','off','on',get_param(gcb,'PlotResponse')};end;set_param(gcb,'MaskVisibilities',visible)|||p7=get_param(gcb,'PlotResponse');if strcmp(p7,'on');visible={'on','on','on','on',get_param(gcb,'Initialize'),get_param(gcb,'Initialize'),'on','on'};else;visible={'on','on','on','on',get_param(gcb,'Initialize'),get_param(gcb,'Initialize'),'on','off'};end;set_param(gcb,'MaskVisibilities',visible)|
      mask Display: plot(X,Y);
  Gain : Gain  Gain=reg(1)  SaturateOnIntegerOverflow=on  OutDataTypeStr=Inherit: Same as input  ParamDataTypeStr=Inherit: Same as input
  Out : Outport
  wires:
  Gain/1 -> 1st order Lowpass/1(In)
  In/1 -> Gain/1
  1st order Lowpass/1(Out) -> Out/1

== system generator_lib/Generator_09152015/GenSet_4MVA_09142015/4MVA Generator with  Primary Controllers/Diesel Engine Speed & Voltage Control fast/Excitation/proportional saturation ==
  Efd : Inport
  Vtf : Inport  Port=2
  Constant : Constant  Value=lim(3)
  Constant1 : Constant  Value=lim(1)
  Constant3 : Constant  Value=0
  Data Type  Conversion{,1..3} (4 alike) : DataTypeConversion  OutDataTypeStr=double  SaturateOnIntegerOverflow=on  RndMeth=Zero
  Logical Operator : Logic
  Logical Operator1 : Logic  Operator=NOT  Inputs=1
  Logical Operator2 : Logic  Operator=NOT  Inputs=1
  Product : Product  SaturateOnIntegerOverflow=on  InputSameDT=on  OutDataTypeStr=Inherit: Same as first input
  Product1 : Product  SaturateOnIntegerOverflow=on  InputSameDT=on  OutDataTypeStr=Inherit: Same as first input
  Product2 : Product  SaturateOnIntegerOverflow=on  InputSameDT=on  OutDataTypeStr=Inherit: Same as first input
  Relational Operator : RelationalOperator  Operator===  InputSameDT=on
  Relational Operator1 : RelationalOperator  Operator=<  InputSameDT=on
  Relational Operator2 : RelationalOperator  Operator=>  InputSameDT=on
  Sum : Sum  SaturateOnIntegerOverflow=on  InputSameDT=on  OutDataTypeStr=Inherit: Same as first input
  Sum1 : Sum  Inputs=+++  SaturateOnIntegerOverflow=on  InputSameDT=on  OutDataTypeStr=Inherit: Same as first input
  Vfdmax : Gain  Gain=lim(2)  SaturateOnIntegerOverflow=on  OutDataTypeStr=Inherit: Same as input  ParamDataTypeStr=Inherit: Same as input
  Vfdmax1 : Gain  Gain=lim(3)  SaturateOnIntegerOverflow=on  OutDataTypeStr=Inherit: Same as input  ParamDataTypeStr=Inherit: Same as input
  Ef : Outport  InitialOutput=0
  wires:
  Vtf/1 -> Vfdmax1/1
  Constant/1 -> Relational Operator/1
  Constant3/1 -> Relational Operator/2
  Vfdmax/1 -> Sum/2
  Vfdmax1/1 -> Sum/1
  Sum/1 -> Product2/2, Relational Operator1/2
  Relational Operator2/1 -> Logical Operator1/1, Logical Operator/1
  Relational Operator1/1 -> Logical Operator2/1, Logical Operator/2
  Constant1/1 -> Relational Operator2/2, Product1/1
  Efd/1 -> Relational Operator2/1, Relational Operator1/1, Product/1
  Sum1/1 -> Ef/1
  Product/1 -> Sum1/1
  Product2/1 -> Sum1/3
  Product1/1 -> Sum1/2
  Logical Operator/1 -> Data Type  Conversion/1
  Data Type  Conversion/1 -> Product/2
  Logical Operator1/1 -> Data Type  Conversion1/1
  Data Type  Conversion1/1 -> Product1/2
  Logical Operator2/1 -> Data Type  Conversion2/1
  Data Type  Conversion2/1 -> Product2/1
  Relational Operator/1 -> Data Type  Conversion3/1
  Data Type  Conversion3/1 -> Vfdmax/1

== system generator_lib/1MVA Generator/GenSet_900kW_07232015/900kW Generator with  Primary Controllers/Diesel Engine Speed & Voltage Control fast/Excitation/Damping kf.s / (tf.s +1)/1st-Order Discrete Filter ==
  In : Inport
  Discrete State-Space : DiscreteStateSpace  A=Ad  B=Bd  C=Cd  D=Dd  X0=x0d  SampleTime=Ts
  Out : Outport  InitialOutput=0
  wires:
  Discrete State-Space/1 -> Out/1
  In/1 -> Discrete State-Space/1

== system generator_lib/1MVA Generator/GenSet_900kW_07232015/900kW Generator with  Primary Controllers/Diesel Engine Speed & Voltage Control fast/Excitation/Exciter  1 / (te.s + ke)/1st order Lowpass ==
  In : Inport
  Discrete State-Space : DiscreteStateSpace  A=Ad  B=Bd  C=Cd  D=Dd  X0=x0d  SampleTime=Ts
  Out : Outport  InitialOutput=0
  wires:
  Discrete State-Space/1 -> Out/1
  In/1 -> Discrete State-Space/1

== system generator_lib/1MVA Generator/GenSet_900kW_07232015/900kW Generator with  Primary Controllers/Diesel Engine Speed & Voltage Control fast/Excitation/Main Regulator ka / (ta.s +1)/1st order Lowpass ==
  In : Inport
  Discrete State-Space : DiscreteStateSpace  A=Ad  B=Bd  C=Cd  D=Dd  X0=x0d  SampleTime=Ts
  Out : Outport  InitialOutput=0
  wires:
  Discrete State-Space/1 -> Out/1
  In/1 -> Discrete State-Space/1

== system generator_lib/Generator_09112015/GenSet_1MVA_09082015/900kW Generator with  Primary Controllers/Diesel Engine Speed & Voltage Control fast/Excitation/Damping kf.s / (tf.s +1)/1st-Order Discrete Filter ==
  In : Inport
  Discrete State-Space : DiscreteStateSpace  A=Ad  B=Bd  C=Cd  D=Dd  X0=x0d  SampleTime=Ts
  Out : Outport  InitialOutput=0
  wires:
  In/1 -> Discrete State-Space/1
  Discrete State-Space/1 -> Out/1
